simulink model "sistema"  (R2025a)
settings: Solver=ode23t  StartTime=0.0  StopTime=10.0  MaxStep=1E-3  RelTol=1e-3
libraries: slpidlib x1, simulink x1
settings DataIOCC: ReturnWorkspaceOutputs=off  TimeSaveName=t
settings DebuggingCC: AlgebraicLoopMsg=none  ArtificialAlgebraicLoopMsg=none  MaxConsecutiveZCsMsg=none

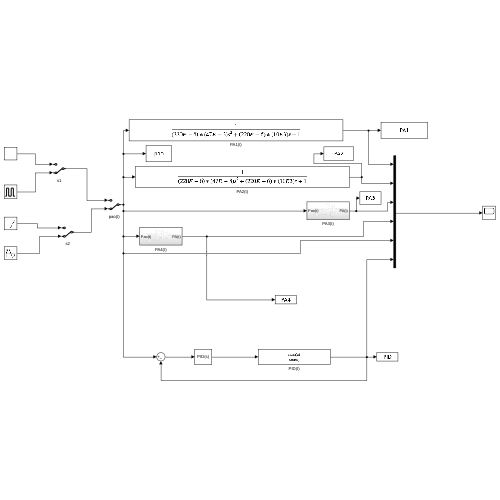
[thumbnail: Simulink's stored preview of the top-level diagram]
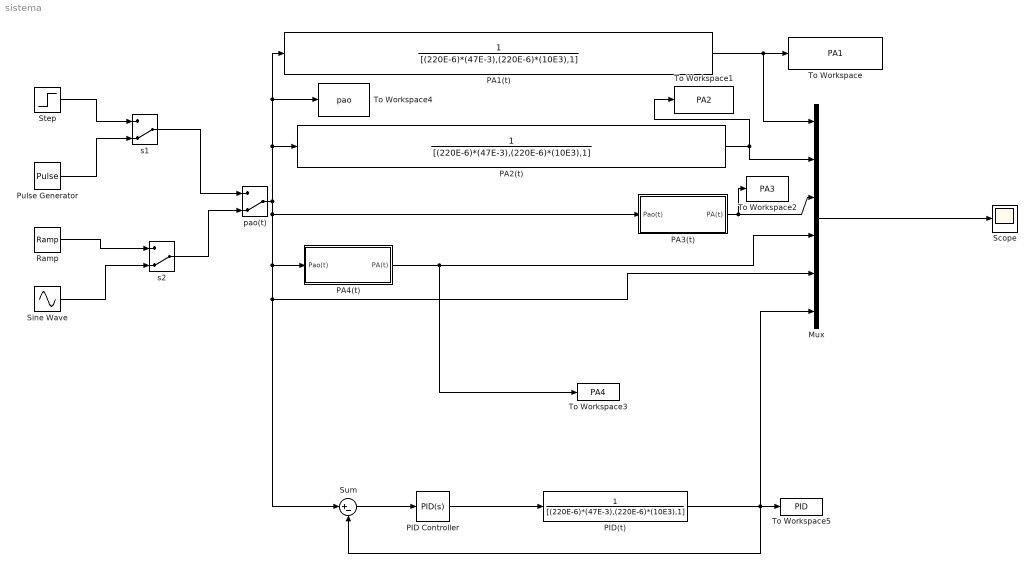
== system sistema ==
  Mux : Mux  Inputs=6
  PA1(t) : TransferFcn  Denominator=[(220E-6)*(47E-3),(220E-6)*(10E3),1]
  PA2(t) : TransferFcn  Denominator=[(220E-6)*(47E-3),(220E-6)*(10E3),1]
  PA3(t) : Subsystem
  PA4(t) : Subsystem
  PID Controller : slpidlib/PID Controller  Controller=PID  Form=Parallel  TimeDomain=Continuous-time  UseExternalTs=off  SampleTime=-1  IntegratorMethod=Forward Euler  FilterMethod=Forward Euler  ControllerParametersSource=internal  P=289.1654  I=7037.5609  UseKiTs=off  D=0.39274  UseExternalDerivativeSource=off  N=502.1982  UseFilter=on  TunerSelectOption=Transfer Function Based (PID Tuner App)  InitialConditionSource=internal  InitialConditionForIntegrator=0  InitialConditionForFilter=0  DifferentiatorICPrevScaledInput=0  ExternalReset=none  TrackingMode=off  Kt=1  LimitOutput=off  SatLimitsSource=internal  UpperSaturationLimit=inf  LowerSaturationLimit=-inf  LinearizeAsGain=on  AntiWindupMode=none  Kb=1  LimitIntegrator=off  UpperIntegratorSaturationLimit=inf  LowerIntegratorSaturationLimit=-inf  POutMin=[]  POutMax=[]  IOutMin=[]  IOutMax=[]  DOutMin=[]  DOutMax=[]  NOutMin=[]  NOutMax=[]  SumOutMin=[]  SumOutMax=[]  SaturationOutMin=[]  SaturationOutMax=[]  PParamMin=[]  PParamMax=[]  IParamMin=[]  IParamMax=[]  DParamMin=[]  DParamMax=[]  NParamMin=[]  NParamMax=[]  KbParamMin=[]  KbParamMax=[]  KtParamMin=[]  KtParamMax=[]  KbOutMin=[]  KbOutMax=[]  KtOutMin=[]  KtOutMax=[]  IntegratorOutMin=[]  IntegratorOutMax=[]  FilterOutMin=[]  FilterOutMax=[]  SumI1OutMin=[]  SumI1OutMax=[]  SumI2OutMin=[]  SumI2OutMax=[]  SumI3OutMin=[]  SumI3OutMax=[]  SumI4OutMin=[]  SumI4OutMax=[]  SumDOutMin=[]  SumDOutMax=[]  DifferentiatorOutMin=[]  DifferentiatorOutMax=[]  FilterDiffOutCoefMin=[]  FilterDiffOutCoefMax=[]  ReciprocalOutMin=[]  ReciprocalOutMax=[]  SumDenOutMin=[]  SumDenOutMax=[]  SumNumOutMin=[]  SumNumOutMax=[]  DivideOutMin=[]  DivideOutMax=[]  UdiffTsProdOutMin=[]  UdiffTsProdOutMax=[]  NTsProdOutMin=[]  NTsProdOutMax=[]  UintegralTsProdOutMin=[]  UintegralTsProdOutMax=[]  UngainTsProdOutMin=[]  UngainTsProdOutMax=[]  ClampingZeroOutDataTypeStr=Inherit: Inherit via back propagation  ClampingZeroOutMin=[]  ClampingZeroOutMax=[]  FilterDenConstantOutDataTypeStr=Inherit: Inherit via back propagation  FilterDenConstantOutMin=[]  FilterDenConstantOutMax=[]  PCopyOutDataTypeStr=Inherit: Inherit via back propagation  PCopyOutMin=[]  PCopyOutMax=[]  NCopyOutDataTypeStr=Inherit: Inherit via back propagation  NCopyOutMin=[]  NCopyOutMax=[]  IntegratorContinuousStateAttributes=''  IntegratorStateMustResolveToSignalObject=off  IntegratorRTWStateStorageClass=Auto  FilterContinuousStateAttributes=''  FilterStateMustResolveToSignalObject=off  FilterRTWStateStorageClass=Auto  ParallelPVariant=InternalParameters  IdealPVariant=Disabled  IVariant=InternalParameters  DVariant=InternalParameters  IntegratorVariant=Continuous  SatVariant=Disabled  AWVariant=Passthrough  PCopyVariant=Disabled  TRVariant=Disabled  FdbkBlocksVariant=Forward  IdealPFdbkVariant=Disabled  SatFdbkVariant=Disabled  DerivativeFilterVariant=ContFilter  NVariant=InternalParameters  NCopyVariant=Disabled  FilterICVariant=InternalICsFilter  IntegratorICVariant=InternalICs  ExternalResetVariant=Disabled  TRSumVariant=Passthrough  SumFdbkVariant=Disabled  SumVariant=Sum_PID  TsampFilterVariant=InternalTs  TsampNgainVariant=Passthrough  TsampIntegralVariant=Disabled_SignalSpec  ExternalSaturationOutDataTypeStr=Inherit: Same as second input  DerivativeSourceVariant=ErrorSignal  PreIntVariant=InternalPreInt
  PID(t) : TransferFcn  Denominator=[(220E-6)*(47E-3),(220E-6)*(10E3),1]
  Pulse Generator : DiscretePulseGenerator  PulseType=Time based  Period=10  PulseWidth=10  PhaseDelay=1
  Ramp : simulink/Sources/Ramp  slope=1/10  start=0  InitialOutput=0
  Scope : Scope
      settings: ActiveDisplayYMinimum=-0.38022024168578028  ActiveDisplayYMaximum=1.2948993090954706
  Sine Wave : Sin  Frequency=pi/2  SampleTime=0
  Step : Step  Time=0  Before=1  SampleTime=0
  Sum : Sum  Inputs=|+-
  To Workspace : ToWorkspace  VariableName=PA1  SampleTime=-1
  To Workspace1 : ToWorkspace  VariableName=PA2  SampleTime=-1
  To Workspace2 : ToWorkspace  VariableName=PA3  SampleTime=-1
  To Workspace3 : ToWorkspace  VariableName=PA4  SampleTime=-1
  To Workspace4 : ToWorkspace  VariableName=pao  SampleTime=-1
  To Workspace5 : ToWorkspace  VariableName=PID  SampleTime=-1
  pao(t) : ManualSwitch  CurrentSetting=0
  s1 : ManualSwitch  CurrentSetting=0
  s2 : ManualSwitch  CurrentSetting=0
  wires:
  Step/1 -> s1/1
  Pulse Generator/1 -> s1/2
  Ramp/1 -> s2/1
  Sine Wave/1 -> s2/2
  s1/1 -> pao(t)/1
  s2/1 -> pao(t)/2
  pao(t)/1 -> Sum/1, Mux/5, PA4(t)/1(Pao(t)), PA3(t)/1(Pao(t)), To Workspace4/1, PA1(t)/1, PA2(t)/1
  PA4(t)/1(PA(t)) -> To Workspace3/1, Mux/4
  PA3(t)/1(PA(t)) -> To Workspace2/1, Mux/3
  PA2(t)/1 -> To Workspace1/1, Mux/2
  Mux/1 -> Scope/1
  PA1(t)/1 -> To Workspace/1, Mux/1
  PID Controller/1 -> PID(t)/1
  Sum/1 -> PID Controller/1
  PID(t)/1 -> To Workspace5/1, Sum/2, Mux/6

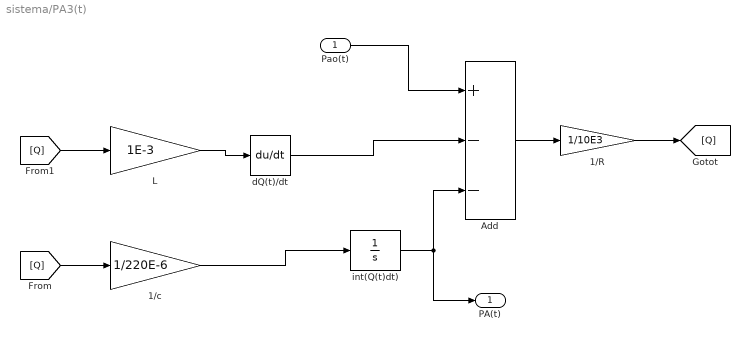
== system sistema/PA3(t) ==
  Pao(t) : Inport
  1/R : Gain  Gain=1/10E3
  1/c : Gain  Gain=1/220E-6
  Add : Sum  Inputs=+--
  L : Gain  Gain=1E-3
  dQ(t)/dt : Derivative
  int(Q(t)dt) : Integrator
  PA(t) : Outport
  wires:
  Add/1 -> 1/R/1
  Pao(t)/1 -> Add/1
  1/R/1 -> [Q]
  int(Q(t)dt)/1 -> PA(t)/1, Add/3
  [Q] -> 1/c/1
  [Q] -> L/1
  L/1 -> dQ(t)/dt/1
  1/c/1 -> int(Q(t)dt)/1
  dQ(t)/dt/1 -> Add/2

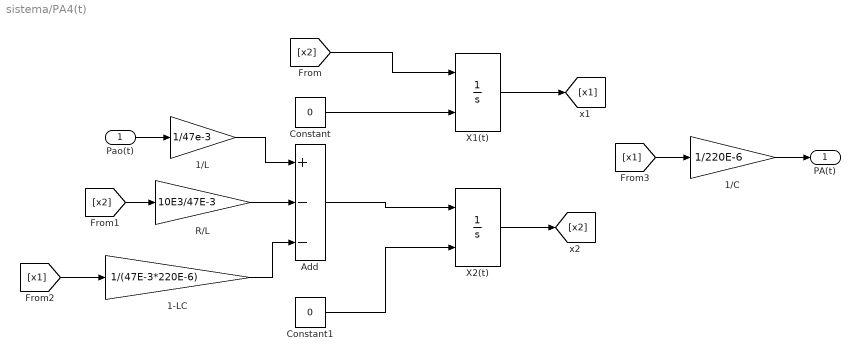
== system sistema/PA4(t) ==
  Pao(t) : Inport
  1-LC : Gain  Gain=1/(47E-3*220E-6)
  1/C : Gain  Gain=1/220E-6
  1/L : Gain  Gain=1/47e-3
  Add : Sum  Inputs=+--
  Constant : Constant  Value=0
  Constant1 : Constant  Value=0
  R/L : Gain  Gain=10E3/47E-3
  X1(t) : Integrator  InitialConditionSource=external
  X2(t) : Integrator  InitialConditionSource=external
  PA(t) : Outport
  wires:
  Constant/1 -> X1(t)/2
  Constant1/1 -> X2(t)/2
  [x2] -> X1(t)/1
  Add/1 -> X2(t)/1
  1/L/1 -> Add/1
  Pao(t)/1 -> 1/L/1
  R/L/1 -> Add/2
  1-LC/1 -> Add/3
  X2(t)/1 -> [x2]
  [x2] -> R/L/1
  [x1] -> 1-LC/1
  X1(t)/1 -> [x1]
  1/C/1 -> PA(t)/1
  [x1] -> 1/C/1
